simulink model "bench_chg"  (R2024b)
settings: Solver=daessc  StartTime=0.0  StopTime=600  MaxStep=0.1  RelTol=1e-3
values from neighbouring files (symbols this model uses):
  P = evalin('base','P')    [audit_aux_chg.m]    (also in audit_axle.m; audit_harness.m; audit_thermal.m; run_bench_aux.m)
  PN = evalin('base','PN')    [run_bench_string_heat.m]
libraries: loco_native_lib x9, fl_lib x4, nesl_utility x3
settings Model: Creator=BillBeverley  LastModifiedBy=BillBeverley

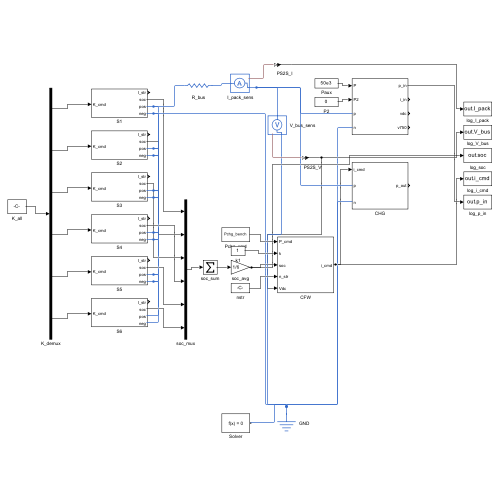
[thumbnail: Simulink's stored preview of the top-level diagram]
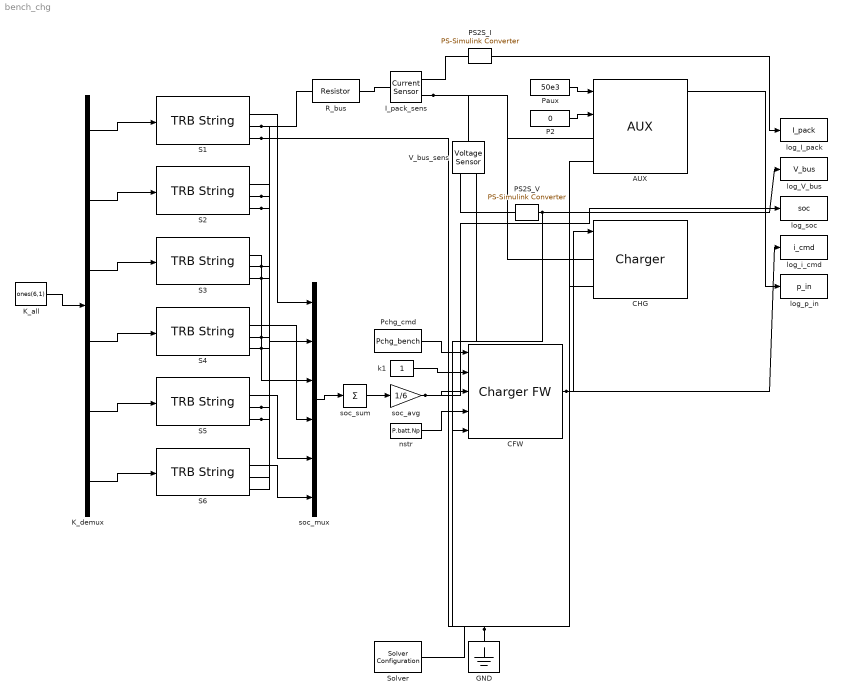
== system bench_chg ==
  AUX : loco_native_lib/AUX  eta=P.aux.eta  P_max=P.aux.P_max  V750=750  V_floor=100
  CFW : loco_native_lib/Charger FW  P_max=P.chg.P_max  I_max=P.chg.I_hw  I_bms=P.chg.I_bms  soc_max=P.chg.soc_max  soc_band=P.chg.soc_band  V_floor=100  N_str_nom=P.batt.Np  Ts=0.01
  CHG : loco_native_lib/Charger  SystemSampleTime=-1  VariantActivationTime=update diagram  AllowFlexibleInterface=on  Latency=0  AutoFrameSizeCalculation=off
  GND : fl_lib/Electrical/Electrical Elements/Electrical Reference
  I_pack_sens : fl_lib/Electrical/Electrical Sensors/Current Sensor
  K_all : Constant  Value=ones(6,1)
  K_demux : Demux  Outputs=6
  P2 : Constant  Value=0
  PS2S_I : nesl_utility/PS-Simulink Converter  PhysicalDomain=network_engine_domain  SubClassName=ps_output  LeftPortType=input  RightPortType=output  PseudoPeriodic=off  Frequencies=[]  VectorFormat=inherit  Unit=A  AffineConversion=off
  PS2S_V : nesl_utility/PS-Simulink Converter  PhysicalDomain=network_engine_domain  SubClassName=ps_output  LeftPortType=input  RightPortType=output  PseudoPeriodic=off  Frequencies=[]  VectorFormat=inherit  Unit=V  AffineConversion=off
  Paux : Constant  Value=50e3
  Pchg_cmd : FromWorkspace  VariableName=Pchg_bench
  R_bus : fl_lib/Electrical/Electrical Elements/Resistor  R=PN.bus.R Ohm  i_specify=off  i_priority=None  i=0 A  i_nominal_specify=off  i_nominal_value=1  i_nominal_unit=A  v_specify=off  v_priority=None  v=0 V  v_nominal_specify=off  v_nominal_value=1  v_nominal_unit=V
  S{1..6} (6 alike) : loco_native_lib/TRB String  SystemSampleTime=-1  VariantActivationTime=update diagram  AllowFlexibleInterface=on  Latency=0  AutoFrameSizeCalculation=off
  Solver : nesl_utility/Solver Configuration  PhysicalDomain=network_engine_domain  SubClassName=solver  LeftPortType=input  RightPortType=generic  Tones=[]  Harmonics=[]  SimulateNoise=off  Profile=off  UseLocalSampling=off  EnableSwitchedLinearOptims=on  FrequencyDomain=off  UseCCode=off  RelTol=0.001  AbsTol=0.001  MinStep=1e-09  ToWorkspace=off  RevertToSquareIcSolve=off  NumHomotopyIterations=100  PhasorMode=off  PhasorModeNumHarmonics=1  ConsistencySolver=NEWTON_XTOL_AFTER_FTOL  IndexReductionMethod=DerivativeReplacement  DoDC=off  ResidualTolerance=1e-09  ConsistencyTolSource=GLOBAL  ConsistencyAbsTol=0.001  ConsistencyRelTol=0.001  ConsistencyTolFactor=0.001  UseLocalSolver=off  LocalSolverChoice=NE_BACKWARD_EULER_ADVANCER  ResolveIndetEquations=on  FunctionEvalNumThread=1  LocalSolverSampleTime=0.001  DoFixedCost=off  MaxNonlinIter=3  MaxModeIter=2  ComputeImpulses=off  ImpulseIterations=2  LinearAlgebra=auto  LinearAlgebraNumThread=0  EquationFormulation=NE_TIME_EF  DelaysMemoryBudget=1024  AutomaticFiltering=on  FilteringTimeConstant=0.001  PartitionStorageMethod=AS_NEEDED  PartitionMemoryBudget=1024  PartitionMethod=ROBUST  MultibodyUseLocalSolver=off  MultibodyLocalSolverChoice=ODE1  MultibodyLocalSolverSampleTime=0.001
  V_bus_sens : fl_lib/Electrical/Electrical Sensors/Voltage Sensor
  k1 : Constant
  log_I_pack : ToWorkspace  VariableName=I_pack  SaveFormat=Timeseries  SampleTime=-1
  log_V_bus : ToWorkspace  VariableName=V_bus  SaveFormat=Timeseries  SampleTime=-1
  log_i_cmd : ToWorkspace  VariableName=i_cmd  SaveFormat=Timeseries  SampleTime=-1
  log_p_in : ToWorkspace  VariableName=p_in  SaveFormat=Timeseries  SampleTime=-1
  log_soc : ToWorkspace  VariableName=soc  SaveFormat=Timeseries  SampleTime=-1
  nstr : Constant  Value=P.batt.Np
  soc_avg : Gain  Gain=1/6
  soc_mux : Mux  Inputs=6
  soc_sum : Sum  Inputs=+
  wires:
  PS2S_I/1 -> log_I_pack/1
  PS2S_V/1 -> log_V_bus/1, CFW/5
  soc_avg/1 -> log_soc/1, CFW/3
  CFW/1 -> log_i_cmd/1, CHG/1
  AUX/1 -> log_p_in/1
  K_all/1 -> K_demux/1
  soc_mux/1 -> soc_sum/1
  soc_sum/1 -> soc_avg/1
  Pchg_cmd/1 -> CFW/1
  k1/1 -> CFW/2
  nstr/1 -> CFW/4
  Paux/1 -> AUX/1
  P2/1 -> AUX/2
  K_demux/1 -> S1/1
  S1/2 -> soc_mux/1
  K_demux/2 -> S2/1
  S2/2 -> soc_mux/2
  K_demux/3 -> S3/1
  S3/2 -> soc_mux/3
  K_demux/4 -> S4/1
  S4/2 -> soc_mux/4
  K_demux/5 -> S5/1
  S5/2 -> soc_mux/5
  K_demux/6 -> S6/1
  S6/2 -> soc_mux/6
  connections:
  R_bus/LConn1 -- S1/RConn1 -- S2/RConn1 -- S3/RConn1 -- S4/RConn1 -- S5/RConn1 -- S6/RConn1
  R_bus/RConn1 -- I_pack_sens/LConn1
  V_bus_sens/LConn1 -- I_pack_sens/RConn2 -- AUX/LConn1 -- CHG/LConn1
  V_bus_sens/RConn2 -- S1/RConn2 -- S2/RConn2 -- S3/RConn2 -- S4/RConn2 -- S5/RConn2 -- S6/RConn2 -- AUX/LConn2 -- CHG/LConn2 -- GND/LConn1 -- Solver/RConn1
  I_pack_sens/RConn1 -- PS2S_I/LConn1
  V_bus_sens/RConn1 -- PS2S_V/LConn1
